simulink model "CLSfixed"  (R2025b)
settings: Solver=FixedStepAuto  StartTime=0.0  StopTime=2000  FixedStep=stepsize  RelTol=1e-3
undefined symbols (not defined in the file or in its folder): AVI, cfg_length, LRI, pNode_length, pPath_length, PVARP, stepsize, URI, VRP
libraries: Libs x14, Libs_unified x9
settings Model: SimulationMode=accelerator  Creator=wai484  LastModifiedBy=rfen801
settings SolverCC: AlgebraicLoopSolver=TrustRegion
settings DataIOCC: ReturnWorkspaceOutputs=off
settings DebuggingCC: UnconnectedInputMsg=warning  UnconnectedOutputMsg=warning  UnconnectedLineMsg=warning  ArithmeticOperatorsInVariantConditions=warning
settings ModelReferenceCC: EnableRefExpFcnMdlSchedulingChecks=on
settings SFSimCC: SimUseLocalCustomCode=off  CustomCodeUndefinedFunction=UseInterfaceOnly
settings RTWCC: RTWUseLocalCustomCode=off  GPUComputeCapability=3.5
settings CodeAppCC: StateflowObjectComments=on

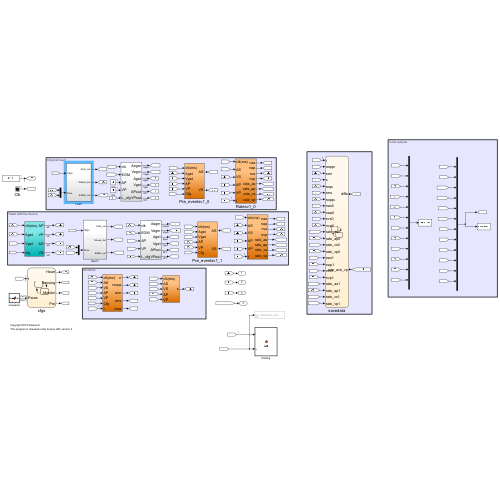
[thumbnail: Simulink's stored preview of the top-level diagram]
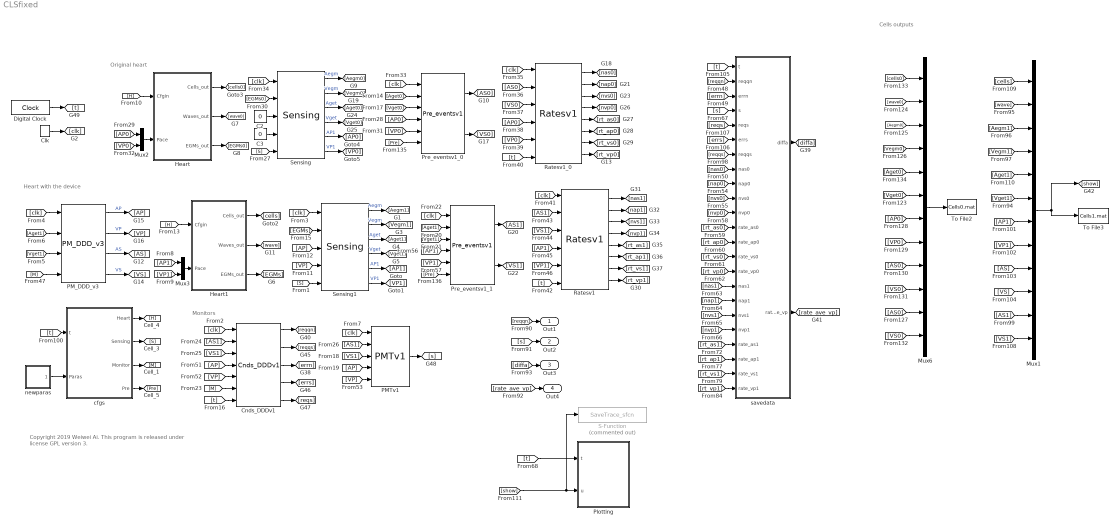
== system CLSfixed ==
  note: Heart with the device
  note: Original heart
  note: Monitors
  note: Copyright 2019 Weiwei Ai.
      | This program is released under license GPL version 3.
  note: Cells outputs
  C2 : Constant  Value=0
  C3 : Constant  Value=0
  Clk : DiscretePulseGenerator  PulseType=Time based  Period=1  PulseWidth=50
  Cnds_DDDv1 : Libs_unified/Cnds_DDDv1  SystemSampleTime=-1  VariantActivationTime=update diagram  EmptyChoice=off  PassThrough=off  PassThroughVariantControl=(default)  EmptyChoiceVariantControl=(default)  AllowFlexibleInterface=on  Latency=0  AutoFrameSizeCalculation=off
  Digital Clock : DigitalClock  SampleTime=stepsize
  Heart : Subsystem
  Heart1 : Subsystem
  Mux1 : Mux  Inputs=12
  Mux2 : Mux  Inputs=2
  Mux3 : Mux  Inputs=2
  Mux6 : Mux  Inputs=12
  PMTv1 : Libs_unified/PMTv1  SystemSampleTime=-1  VariantActivationTime=update diagram  EmptyChoice=off  PassThrough=off  PassThroughVariantControl=(default)  EmptyChoiceVariantControl=(default)  AllowFlexibleInterface=on  Latency=0  AutoFrameSizeCalculation=off
  PM_DDD_v3 : Libs_unified/PM_DDD_v3  SystemSampleTime=-1  VariantActivationTime=update diagram  EmptyChoice=off  PassThrough=off  PassThroughVariantControl=(default)  EmptyChoiceVariantControl=(default)  AllowFlexibleInterface=on  Latency=0  AutoFrameSizeCalculation=off
  Plotting : MATLAB Function  TreatAsAtomicUnit=on  SystemSampleTime=stepsize*5
  Pre_eventsv1_0 : Libs_unified/Pre_eventsv1  SystemSampleTime=-1  VariantActivationTime=update diagram  EmptyChoice=off  PassThrough=off  PassThroughVariantControl=(default)  EmptyChoiceVariantControl=(default)  AllowFlexibleInterface=on  Latency=0  AutoFrameSizeCalculation=off
  Pre_eventsv1_1 : Libs_unified/Pre_eventsv1  SystemSampleTime=-1  VariantActivationTime=update diagram  EmptyChoice=off  PassThrough=off  PassThroughVariantControl=(default)  EmptyChoiceVariantControl=(default)  AllowFlexibleInterface=on  Latency=0  AutoFrameSizeCalculation=off
  Ratesv1 : Libs_unified/Ratesv1  SystemSampleTime=-1  VariantActivationTime=update diagram  EmptyChoice=off  PassThrough=off  PassThroughVariantControl=(default)  EmptyChoiceVariantControl=(default)  AllowFlexibleInterface=on  Latency=0  AutoFrameSizeCalculation=off
  Ratesv1_0 : Libs_unified/Ratesv1  SystemSampleTime=-1  VariantActivationTime=update diagram  EmptyChoice=off  PassThrough=off  PassThroughVariantControl=(default)  EmptyChoiceVariantControl=(default)  AllowFlexibleInterface=on  Latency=0  AutoFrameSizeCalculation=off
  S-Function : S-Function  Commented=on  FunctionName=SaveTrace_sfcn  Parameters=1  SFunctionDeploymentMode=off  EnableBusSupport=off
  Sensing : Libs_unified/Sensing  SystemSampleTime=-1  VariantActivationTime=update diagram  EmptyChoice=off  PassThrough=off  PassThroughVariantControl=(default)  EmptyChoiceVariantControl=(default)  AllowFlexibleInterface=on  Latency=0  AutoFrameSizeCalculation=off
  Sensing1 : Libs_unified/Sensing  SystemSampleTime=-1  VariantActivationTime=update diagram  EmptyChoice=off  PassThrough=off  PassThroughVariantControl=(default)  EmptyChoiceVariantControl=(default)  AllowFlexibleInterface=on  Latency=0  AutoFrameSizeCalculation=off
  To File2 : ToFile  Filename=Cells0.mat  MatrixName=cells
      settings: Decimation=2
  To File3 : ToFile  Filename=Cells1.mat  MatrixName=cells
      settings: Decimation=2
  cfgs : Stateflow chart  TreatAsAtomicUnit=on
  newparas : MATLAB Function  TreatAsAtomicUnit=on
  savedata : Stateflow chart  TreatAsAtomicUnit=on
  Out1 : Outport
  Out2 : Outport  Port=2
  Out3 : Outport  Port=3
  Out4 : Outport  Port=4
  wires:
  [M] -> PM_DDD_v3/4
  Clk/1 -> [clk]
  [clk] -> PM_DDD_v3/1
  [Aget1] -> PM_DDD_v3/2
  [Vget1] -> PM_DDD_v3/3
  Heart1/1(Cells_out) -> [cells]
  Heart1/2(Waves_out) -> [wave]
  Heart1/3(EGMs_out) -> [EGMs]
  cfgs/1(Heart) -> [H]
  cfgs/2(Sensing) -> [S]
  PM_DDD_v3/1 -> [AP]  "AP"
  PM_DDD_v3/2 -> [VP]  "VP"
  PM_DDD_v3/3 -> [AS]  "AS"
  PM_DDD_v3/4 -> [VS]  "VS"
  [AP1] -> Mux3/1
  [VP1] -> Mux3/2
  Sensing1/1 -> [Aegm1]  "Aegm"
  Sensing1/2 -> [Vegm1]  "Vegm"
  Sensing1/3 -> [Aget1]  "Aget"
  Sensing1/4 -> [Vget1]  "Vget"
  Sensing1/5 -> [AP1]  "AP1"
  Sensing1/6 -> [VP1]  "VP1"
  [clk] -> Pre_eventsv1_1/1
  [Aget1] -> Pre_eventsv1_1/2
  [Vget1] -> Pre_eventsv1_1/3
  [AP1] -> Pre_eventsv1_1/4
  [VP1] -> Pre_eventsv1_1/5
  [Pre] -> Pre_eventsv1_1/6
  Pre_eventsv1_1/1 -> [AS1]
  Pre_eventsv1_1/2 -> [VS1]
  cfgs/3(Monitor) -> [M]
  newparas/1(newparas) -> cfgs/2(Paras)
  Heart/1(Cells_out) -> [cells0]
  Heart/2(Waves_out) -> [wave0]
  Heart/3(EGMs_out) -> [EGMs0]
  [AP0] -> Mux2/1
  [H] -> Heart/1(Cfgin)
  Mux2/1 -> Heart/2(Pace)
  Sensing/1 -> [Aegm0]  "Aegm"
  Sensing/2 -> [Vegm0]  "Vegm"
  Sensing/3 -> [Aget0]  "Aget"
  Sensing/4 -> [Vget0]  "Vget"
  Sensing/5 -> [AP0]  "AP1"
  Sensing/6 -> [VP0]  "VP1"
  [clk] -> Pre_eventsv1_0/1
  [Aget0] -> Pre_eventsv1_0/2
  [Vget0] -> Pre_eventsv1_0/3
  [AP0] -> Pre_eventsv1_0/4
  [Pre] -> Pre_eventsv1_0/6
  Pre_eventsv1_0/1 -> [AS0]
  Pre_eventsv1_0/2 -> [VS0]
  [VP0] -> Pre_eventsv1_0/5
  [VP0] -> Mux2/2
  [clk] -> Sensing/1
  [S] -> Sensing/5
  C3/1 -> Sensing/4
  C2/1 -> Sensing/3
  [EGMs0] -> Sensing/2
  [clk] -> Sensing1/1
  [EGMs] -> Sensing1/2
  [AP] -> Sensing1/3
  [VP] -> Sensing1/4
  [S] -> Sensing1/5
  Digital Clock/1 -> [t]
  [t] -> cfgs/1(t)
  cfgs/4(Pre) -> [Pre]
  [clk] -> Ratesv1_0/1
  [AS0] -> Ratesv1_0/2
  [VS0] -> Ratesv1_0/3
  [AP0] -> Ratesv1_0/4
  [VP0] -> Ratesv1_0/5
  [t] -> Ratesv1_0/6
  Ratesv1_0/1 -> [nas0]
  Ratesv1_0/2 -> [nap0]
  Ratesv1_0/3 -> [nvs0]
  Ratesv1_0/4 -> [nvp0]
  Ratesv1_0/5 -> [rt_as0]
  Ratesv1_0/6 -> [rt_ap0]
  Ratesv1_0/7 -> [rt_vs0]
  Ratesv1_0/8 -> [rt_vp0]
  [clk] -> Ratesv1/1
  [t] -> Ratesv1/6
  Ratesv1/1 -> [nas1]
  Ratesv1/2 -> [nap1]
  Ratesv1/3 -> [nvs1]
  Ratesv1/4 -> [nvp1]
  Ratesv1/5 -> [rt_as1]
  Ratesv1/6 -> [rt_ap1]
  Ratesv1/7 -> [rt_vs1]
  Ratesv1/8 -> [rt_vp1]
  [AS1] -> Ratesv1/2
  [VS1] -> Ratesv1/3
  [AP1] -> Ratesv1/4
  [VP1] -> Ratesv1/5
  Cnds_DDDv1/1 -> [reqqn]
  Cnds_DDDv1/2 -> [reqqs]
  Cnds_DDDv1/5 -> [reqs]
  [AP] -> PMTv1/4
  [VP] -> PMTv1/5
  [AS1] -> Cnds_DDDv1/2
  [VS1] -> Cnds_DDDv1/3
  [AP] -> Cnds_DDDv1/4
  [VP] -> Cnds_DDDv1/5
  [M] -> Cnds_DDDv1/6
  [t] -> Cnds_DDDv1/7
  Cnds_DDDv1/4 -> [errs]
  Cnds_DDDv1/3 -> [errn]
  [clk] -> Cnds_DDDv1/1
  PMTv1/1 -> [s]
  [VS1] -> PMTv1/3
  [AS1] -> PMTv1/2
  [clk] -> PMTv1/1
  [t] -> savedata/1(t)
  [reqqn] -> savedata/2(reqqn)
  [errn] -> savedata/3(errn)
  [s] -> savedata/4(s)
  [errs] -> savedata/6(errs)
  [reqs] -> savedata/5(reqs)
  [reqqs] -> savedata/7(reqqs)
  [nas0] -> savedata/8(nas0)
  [nap0] -> savedata/9(nap0)
  [nvs0] -> savedata/10(nvs0)
  [nvp0] -> savedata/11(nvp0)
  [rt_as0] -> savedata/12(rate_as0)
  [rt_ap0] -> savedata/13(rate_ap0)
  [rt_vs0] -> savedata/14(rate_vs0)
  [rt_vp0] -> savedata/15(rate_vp0)
  [nas1] -> savedata/16(nas1)
  [nap1] -> savedata/17(nap1)
  [nvs1] -> savedata/18(nvs1)
  [nvp1] -> savedata/19(nvp1)
  [rt_as1] -> savedata/20(rate_as1)
  [rt_ap1] -> savedata/21(rate_ap1)
  [rt_vs1] -> savedata/22(rate_vs1)
  [rt_vp1] -> savedata/23(rate_vp1)
  savedata/1(diffa) -> [diffa]
  savedata/2(rate_ave_vp) -> [rate_ave_vp]
  [reqqn] -> Out1/1
  [s] -> Out2/1
  [diffa] -> Out3/1
  [rate_ave_vp] -> Out4/1
  [wave0] -> Mux6/2
  [Aegm0] -> Mux6/3
  [Vegm0] -> Mux6/4
  [cells0] -> Mux6/1
  [Aget0] -> Mux6/5
  [Vget0] -> Mux6/6
  [AP0] -> Mux6/7
  [VP0] -> Mux6/8
  [AS0] -> Mux6/9
  [VS0] -> Mux6/10
  [AS0] -> Mux6/11
  [VS0] -> Mux6/12
  [wave] -> Mux1/2
  [Aegm1] -> Mux1/3
  [Vegm1] -> Mux1/4
  [cells] -> Mux1/1
  [Aget1] -> Mux1/5
  [Vget1] -> Mux1/6
  [AP1] -> Mux1/7
  [VP1] -> Mux1/8
  [AS] -> Mux1/9
  [VS] -> Mux1/10
  [AS1] -> Mux1/11
  [VS1] -> Mux1/12
  Mux6/1 -> To File2/1
  Mux1/1 -> To File3/1, [show]
  [show] -> S-Function/1, Plotting/2(u)
  [t] -> Plotting/1(t)
  Mux3/1 -> Heart1/2(Pace)
  [H] -> Heart1/1(Cfgin)

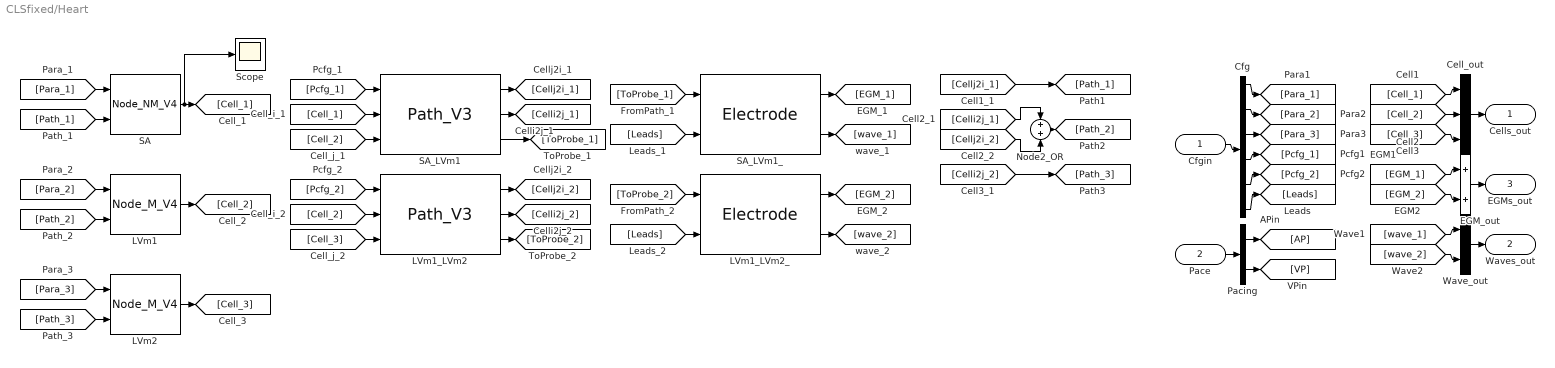
== system CLSfixed/Heart ==
  Cfgin : Inport
  Pace : Inport  Port=2
  Cell_out : Mux  Inputs=3
  Cfg : Demux  Outputs=[23,25,25,11,11,28]
  EGM_out : Sum  Inputs=2
  LVm1 : Libs/Node_M_V4  SystemSampleTime=-1  VariantActivationTime=update diagram  EmptyChoice=off  PassThrough=off  PassThroughVariantControl=(default)  EmptyChoiceVariantControl=(default)  AllowFlexibleInterface=on  Latency=0  AutoFrameSizeCalculation=off
  LVm1_LVm2 : Libs/Path_V3  SystemSampleTime=-1  VariantActivationTime=update diagram  EmptyChoice=off  PassThrough=off  PassThroughVariantControl=(default)  EmptyChoiceVariantControl=(default)  AllowFlexibleInterface=on  Latency=0  AutoFrameSizeCalculation=off
  LVm1_LVm2_ : Libs/Electrode  SystemSampleTime=-1  VariantActivationTime=update diagram  EmptyChoice=off  PassThrough=off  PassThroughVariantControl=(default)  EmptyChoiceVariantControl=(default)  AllowFlexibleInterface=on  Latency=0  AutoFrameSizeCalculation=off
  LVm2 : Libs/Node_M_V4  SystemSampleTime=-1  VariantActivationTime=update diagram  EmptyChoice=off  PassThrough=off  PassThroughVariantControl=(default)  EmptyChoiceVariantControl=(default)  AllowFlexibleInterface=on  Latency=0  AutoFrameSizeCalculation=off
  Node2_OR : Sum  Inputs=2
  Pacing : Demux  Outputs=2
  SA : Libs/Node_NM_V4  SystemSampleTime=-1  VariantActivationTime=update diagram  EmptyChoice=off  PassThrough=off  PassThroughVariantControl=(default)  EmptyChoiceVariantControl=(default)  AllowFlexibleInterface=on  Latency=0  AutoFrameSizeCalculation=off
  SA_LVm1 : Libs/Path_V3  SystemSampleTime=-1  VariantActivationTime=update diagram  EmptyChoice=off  PassThrough=off  PassThroughVariantControl=(default)  EmptyChoiceVariantControl=(default)  AllowFlexibleInterface=on  Latency=0  AutoFrameSizeCalculation=off
  SA_LVm1_ : Libs/Electrode  SystemSampleTime=-1  VariantActivationTime=update diagram  EmptyChoice=off  PassThrough=off  PassThroughVariantControl=(default)  EmptyChoiceVariantControl=(default)  AllowFlexibleInterface=on  Latency=0  AutoFrameSizeCalculation=off
  Scope : Scope
  Wave_out : Mux  Inputs=2
  Cells_out : Outport
  Waves_out : Outport  Port=2
  EGMs_out : Outport  Port=3
  wires:
  [wave_2] -> Wave_out/2
  [wave_1] -> Wave_out/1
  [EGM_2] -> EGM_out/2
  [EGM_1] -> EGM_out/1
  [Cell_3] -> Cell_out/3
  [Cell_2] -> Cell_out/2
  [Cell_1] -> Cell_out/1
  Wave_out/1 -> Waves_out/1
  EGM_out/1 -> EGMs_out/1
  Cell_out/1 -> Cells_out/1
  Pacing/2 -> [VP]
  Pacing/1 -> [AP]
  Cfg/6 -> [Leads]
  Cfg/5 -> [Pcfg_2]
  Cfg/4 -> [Pcfg_1]
  Cfg/3 -> [Para_3]
  Cfg/2 -> [Para_2]
  Cfg/1 -> [Para_1]
  Pace/1 -> Pacing/1
  Cfgin/1 -> Cfg/1
  [Celli2j_2] -> [Path_3]
  Node2_OR/1 -> [Path_2]
  [Cellj2i_2] -> Node2_OR/2
  [Celli2j_1] -> Node2_OR/1
  [Cellj2i_1] -> [Path_1]
  [Leads] -> LVm1_LVm2_/2
  [ToProbe_2] -> LVm1_LVm2_/1
  LVm1_LVm2_/2 -> [wave_2]
  LVm1_LVm2_/1 -> [EGM_2]
  [Leads] -> SA_LVm1_/2
  [ToProbe_1] -> SA_LVm1_/1
  SA_LVm1_/2 -> [wave_1]
  SA_LVm1_/1 -> [EGM_1]
  [Cell_3] -> LVm1_LVm2/3
  [Cell_2] -> LVm1_LVm2/2
  [Pcfg_2] -> LVm1_LVm2/1
  LVm1_LVm2/3 -> [ToProbe_2]
  LVm1_LVm2/2 -> [Celli2j_2]
  LVm1_LVm2/1 -> [Cellj2i_2]
  [Cell_2] -> SA_LVm1/3
  [Cell_1] -> SA_LVm1/2
  [Pcfg_1] -> SA_LVm1/1
  SA_LVm1/3 -> [ToProbe_1]
  SA_LVm1/2 -> [Celli2j_1]
  SA_LVm1/1 -> [Cellj2i_1]
  [Path_3] -> LVm2/2
  [Para_3] -> LVm2/1
  LVm2/1 -> [Cell_3]
  [Path_2] -> LVm1/2
  [Para_2] -> LVm1/1
  LVm1/1 -> [Cell_2]
  [Path_1] -> SA/2
  [Para_1] -> SA/1
  SA/1 -> Scope/1, [Cell_1]

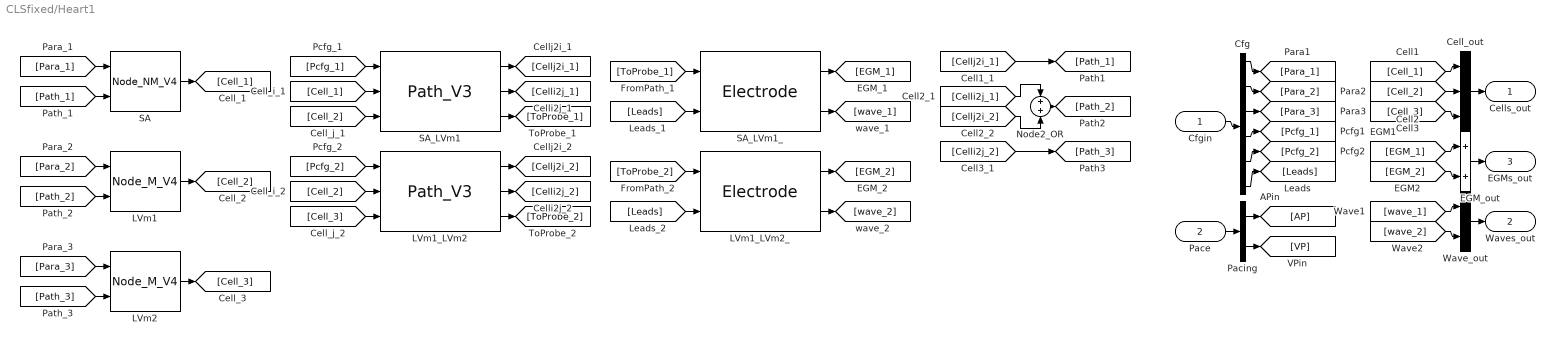
== system CLSfixed/Heart1 ==
  Cfgin : Inport
  Pace : Inport  Port=2
  Cell_out : Mux  Inputs=3
  Cfg : Demux  Outputs=[23,25,25,11,11,28]
  EGM_out : Sum  Inputs=2
  LVm1 : Libs/Node_M_V4  SystemSampleTime=-1  VariantActivationTime=update diagram  EmptyChoice=off  PassThrough=off  PassThroughVariantControl=(default)  EmptyChoiceVariantControl=(default)  AllowFlexibleInterface=on  Latency=0  AutoFrameSizeCalculation=off
  LVm1_LVm2 : Libs/Path_V3  SystemSampleTime=-1  VariantActivationTime=update diagram  EmptyChoice=off  PassThrough=off  PassThroughVariantControl=(default)  EmptyChoiceVariantControl=(default)  AllowFlexibleInterface=on  Latency=0  AutoFrameSizeCalculation=off
  LVm1_LVm2_ : Libs/Electrode  SystemSampleTime=-1  VariantActivationTime=update diagram  EmptyChoice=off  PassThrough=off  PassThroughVariantControl=(default)  EmptyChoiceVariantControl=(default)  AllowFlexibleInterface=on  Latency=0  AutoFrameSizeCalculation=off
  LVm2 : Libs/Node_M_V4  SystemSampleTime=-1  VariantActivationTime=update diagram  EmptyChoice=off  PassThrough=off  PassThroughVariantControl=(default)  EmptyChoiceVariantControl=(default)  AllowFlexibleInterface=on  Latency=0  AutoFrameSizeCalculation=off
  Node2_OR : Sum  Inputs=2
  Pacing : Demux  Outputs=2
  SA : Libs/Node_NM_V4  SystemSampleTime=-1  VariantActivationTime=update diagram  EmptyChoice=off  PassThrough=off  PassThroughVariantControl=(default)  EmptyChoiceVariantControl=(default)  AllowFlexibleInterface=on  Latency=0  AutoFrameSizeCalculation=off
  SA_LVm1 : Libs/Path_V3  SystemSampleTime=-1  VariantActivationTime=update diagram  EmptyChoice=off  PassThrough=off  PassThroughVariantControl=(default)  EmptyChoiceVariantControl=(default)  AllowFlexibleInterface=on  Latency=0  AutoFrameSizeCalculation=off
  SA_LVm1_ : Libs/Electrode  SystemSampleTime=-1  VariantActivationTime=update diagram  EmptyChoice=off  PassThrough=off  PassThroughVariantControl=(default)  EmptyChoiceVariantControl=(default)  AllowFlexibleInterface=on  Latency=0  AutoFrameSizeCalculation=off
  Wave_out : Mux  Inputs=2
  Cells_out : Outport
  Waves_out : Outport  Port=2
  EGMs_out : Outport  Port=3
  wires:
  [wave_2] -> Wave_out/2
  [wave_1] -> Wave_out/1
  [EGM_2] -> EGM_out/2
  [EGM_1] -> EGM_out/1
  [Cell_3] -> Cell_out/3
  [Cell_2] -> Cell_out/2
  [Cell_1] -> Cell_out/1
  Wave_out/1 -> Waves_out/1
  EGM_out/1 -> EGMs_out/1
  Cell_out/1 -> Cells_out/1
  Pacing/2 -> [VP]
  Pacing/1 -> [AP]
  Cfg/6 -> [Leads]
  Cfg/5 -> [Pcfg_2]
  Cfg/4 -> [Pcfg_1]
  Cfg/3 -> [Para_3]
  Cfg/2 -> [Para_2]
  Cfg/1 -> [Para_1]
  Pace/1 -> Pacing/1
  Cfgin/1 -> Cfg/1
  [Celli2j_2] -> [Path_3]
  Node2_OR/1 -> [Path_2]
  [Cellj2i_2] -> Node2_OR/2
  [Celli2j_1] -> Node2_OR/1
  [Cellj2i_1] -> [Path_1]
  [Leads] -> LVm1_LVm2_/2
  [ToProbe_2] -> LVm1_LVm2_/1
  LVm1_LVm2_/2 -> [wave_2]
  LVm1_LVm2_/1 -> [EGM_2]
  [Leads] -> SA_LVm1_/2
  [ToProbe_1] -> SA_LVm1_/1
  SA_LVm1_/2 -> [wave_1]
  SA_LVm1_/1 -> [EGM_1]
  [Cell_3] -> LVm1_LVm2/3
  [Cell_2] -> LVm1_LVm2/2
  [Pcfg_2] -> LVm1_LVm2/1
  LVm1_LVm2/3 -> [ToProbe_2]
  LVm1_LVm2/2 -> [Celli2j_2]
  LVm1_LVm2/1 -> [Cellj2i_2]
  [Cell_2] -> SA_LVm1/3
  [Cell_1] -> SA_LVm1/2
  [Pcfg_1] -> SA_LVm1/1
  SA_LVm1/3 -> [ToProbe_1]
  SA_LVm1/2 -> [Celli2j_1]
  SA_LVm1/1 -> [Cellj2i_1]
  [Path_3] -> LVm2/2
  [Para_3] -> LVm2/1
  LVm2/1 -> [Cell_3]
  [Path_2] -> LVm1/2
  [Para_2] -> LVm1/1
  LVm1/1 -> [Cell_2]
  [Path_1] -> SA/2
  [Para_1] -> SA/1
  SA/1 -> [Cell_1]

== matlab function CLSfixed/Plotting ==
  data: t input; u input
function fcn(t,u)
%coder.extrinsic('evalin')
coder.extrinsic('updateGUIplots')
fun = 'updateGUIplots';
updateGUIplots(t,u)
%feval(fun,t,u)
end

== stateflow chart CLSfixed/cfgs ==
  settings: executeAtInitialization=1
  state Ini
  state wait
  Ini -> wait : [t>800]{pUpdate(Paras);}
  (default) -> Ini : {Sensing=Scfgf;[Monitor, Pre]=Precfg;...
      |  [Heart] =LoadInit;}
  data: Scfg function_output; Mcfg function_output; Preout function_output; LRI parameter; AVI parameter; VRP parameter; URI parameter; PVARP parameter; Parasin function_input; pNode_length parameter; pPath_length parameter; Hcfg function_output; cfg_length parameter; Heart output; Sensing output; Monitor output; t input; Paras input; Pre output
  function Scfg= Scfgf:
    | function Scfg= Scfgf
    | 
    | %% desired
    | xa=1;
    | xc=0.05;
    | xc1=0.1;
    | xd=1;
    | xe=0.1;
    | avd=100;
    | vad=100;
    | uni_a=1;
    | Sens_a=0.6;
    | Amp_ap=500;
    | uni_v=1;
    | Sens_v=2.8;
    | Amp_vp=500;
    | 
    | Scfg=[xa xc xc1 xd xe avd vad uni_a Sens_a Amp_ap uni_v Sens_v Amp_vp]';
    | 
    | end
  function [Mcfg,Preout]= Precfg:
    | function [Mcfg,Preout]= Precfg
    | % 
    | % LRI=1000;
    | % AVI=170;
    | % URI=500;
    | % VRP=230;
    | % PVARP=250;
    | Mcfg=[LRI AVI URI VRP PVARP];
    | Preout=[VRP PVARP];
    | 
    | end
  function pUpdate(Parasin):
    | %% Get the index of the parameter
    | function pUpdate(Parasin)
    | %#codegen
    | coder.extrinsic('evalin');
    | coder.extrinsic('assignin');
    | Nodein=zeros(1,pNode_length); % The total number of cell cfg ports
    | Nodein=evalin('base', 'pNode');
    | Pathin=zeros(1,pPath_length); % The total number of path cfg ports
    | Pathin=evalin('base', 'pPath');
    | for n=1:pNode_length
    |     m=Nodein(n);
    |     Heart(m)=Parasin(n);
    | end
    | 
    | for n=1:pPath_length
    |     m=Pathin(n);
    |     nn=n+length(Nodein);
    |     Heart(m)=Parasin(nn);
    | end
    | 
    | assignin('base', 'Params', Parasin);
    | 
    | end
  function Hcfg   = LoadInit:
    | function Hcfg   = LoadInit
    | %#codegen
    | coder.extrinsic('evalin');
    | Hcfg1=zeros(1,cfg_length); % The total number of cfg ports
    | Hcfg1=evalin('base', 'cfgdata');
    | Hcfg=Hcfg1';
    | end

== matlab function CLSfixed/newparas ==
  data: newparas output; paras_length parameter

function newparas= auto(paras_length)

coder.extrinsic('evalin');
%par_length = evalin('base','paras_length')
newparas=zeros(1,paras_length); % The total number of cell cfg ports
newparas=evalin('base', 'pp');

end

== stateflow chart CLSfixed/savedata ==
  settings: executeAtInitialization=1
  state termi
  state difa
  state Ini
  difa -> termi [order 1] : [rate_ave_a0>=60]/{coder.extrinsic('assignin');diffa=rate_ave_a1-rate_ave_a0;assignin('base', 'diffa', diffa);}
  (default) -> Ini : {rate_ave_vp=0; diffa=0;smax=0;}
  Ini -> difa [order 1] : [t>=29998]{coder.extrinsic('assignin','mean');assignin('base', 'reqqn', reqqn);assignin('base', 'errn', errn);assignin('base', 'smax', smax);...
      | assignin('base', 'errs', errs);assignin('base', 'reqs', reqs);assignin('base', 'reqqs', reqqs);...
      | assignin('base', 'nas0', nas0);assignin('base', 'nap0', nap0);assignin('base', 'nvs0', nvs0);assignin('base', 'nvp0', nvp0);...
      | assignin('base', 'rate_as0', rate_as0);assignin('base', 'rate_ap0', rate_ap0);assignin('base', 'rate_vs0', rate_vs0);assignin('base', 'rate_vp0', rate_vp0);...
      | assignin('base', 'nas1', nas1);assignin('base', 'nap1', nap1);assignin('base', 'nvs1', nvs1);assignin('base', 'nvp1', nvp1);...
      | assignin('base', 'rate_as1', rate_as1);assignin('base', 'rate_ap1', rate_ap1);assignin('base', 'rate_vs1', rate_vs1);assignin('base', 'rate_vp1', rate_vp1);...
      | rate_ave_vp=mean(rate_vp1(2,1:nvp1));assignin('base', 'rate_ave_vp', rate_ave_vp);...
      | rate_ave_a1=0;rate_ave_a1=mean([rate_as1(2,1:nas1) ]);rate_ave_a0=0;rate_ave_a0=mean(rate_as0(2,1:nas0));}
  difa -> termi [order 2] : [rate_ave_a0<60]/{coder.extrinsic('assignin');diffa=rate_ave_a1-60;assignin('base', 'diffa', diffa);}
  Ini -> Ini [order 2] : [s>smax]/{smax=s;}
  data: t input; reqqn input; errn input; s input; reqs input; errs input; reqqs input; nas0 input; nap0 input; nvs0 input; nvp0 input; rate_as0 input; rate_ap0 input; rate_vs0 input; rate_vp0 input; nas1 input; nap1 input; nvs1 input; nvp1 input; rate_as1 input; rate_ap1 input; rate_vs1 input; rate_vp1 input; diffa output double; rate_ave_a1 local double; rate_ave_vp output double; rate_ave_a0 local double; smax local
